simulink model "kalman_direction_updater"  (R2014a)
settings: Solver=FixedStepDiscrete  StartTime=0.0  StopTime=t_sim  FixedStep=t_step  RelTol=1e-3
undefined symbols (not defined in the file): omega_B
libraries: lib_gyro_fusion x7, vrlib x1
settings Model: Creator=kirill  LastModifiedBy=kirill

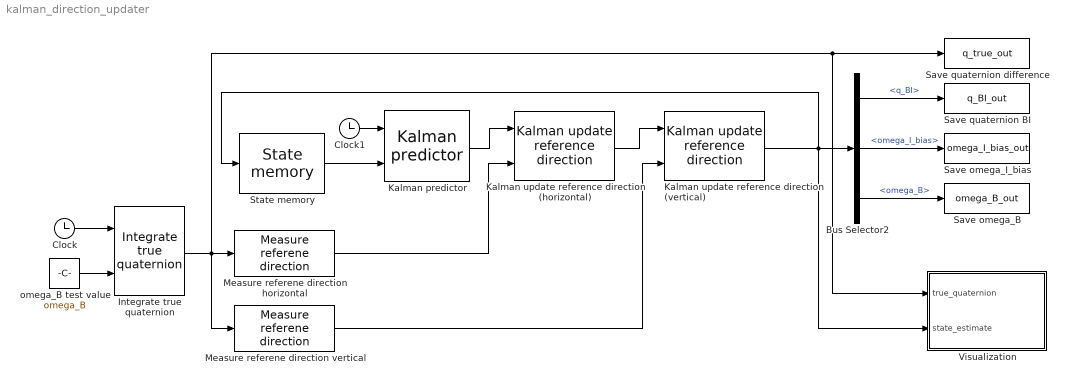
== system kalman_direction_updater ==
  Bus Selector2 : BusSelector  OutputSignals=q_BI,omega_I_bias,omega_B
  Clock : Clock
  Clock1 : Clock
  Integrate true quaternion : lib_gyro_fusion/Integrate true quaternion  q_BI_init=q_init
  Kalman predictor : lib_gyro_fusion/Kalman predictor  q_noise=q_noise  omega_B_noise=omega_B_noise  omega_I_bias_noise=omega_bias_I_noise
  Kalman update reference direction (horizontal) : lib_gyro_fusion/Kalman update reference direction
  Kalman update reference direction (vertical) : lib_gyro_fusion/Kalman update reference direction
  Measure referene direction horizontal : lib_gyro_fusion/Measure referene direction  ref_direction=horizontal_direction  measurement_noise_power=horizontal_direction_noise_power  measurement_sample_rate=t_step  source_seeds=horizontal_direction_seeds  R_direction=horizontal_direction_R
  Measure referene direction vertical : lib_gyro_fusion/Measure referene direction  ref_direction=vertical_direction  measurement_noise_power=vertical_direction_noise_power  measurement_sample_rate=t_step  source_seeds=vertical_direction_seeds  R_direction=vertical_direction_R
  Save omega_B : ToWorkspace  VariableName=omega_B_out  SaveFormat=Timeseries  SampleTime=-1
  Save omega_I_bias : ToWorkspace  VariableName=omega_I_bias_out  SaveFormat=Timeseries  SampleTime=-1
  Save quaternion BI : ToWorkspace  VariableName=q_BI_out  SaveFormat=Timeseries  SampleTime=-1
  Save quaternion difference : ToWorkspace  VariableName=q_true_out  SaveFormat=Timeseries  SampleTime=-1
  State memory : lib_gyro_fusion/State memory  q_BI_init=[1; 0; 0; 0]  omega_B_init=[0; 0; 0]  omega_I_bias_init=[0; 0; 0]  P_full_init=eye(9)
  Visualization : Subsystem
  omega_B test value : Constant  Value=omega_B
  wires:
  State memory/1 -> Kalman predictor/2
  Clock/1 -> Integrate true quaternion/1
  Integrate true quaternion/1 -> Measure referene direction horizontal/1, Measure referene direction vertical/1, Visualization/1(true_quaternion), Save quaternion difference/1
  omega_B test value/1 -> Integrate true quaternion/2
  Bus Selector2/2 -> Save omega_I_bias/1  "<omega_I_bias>"
  Bus Selector2/3 -> Save omega_B/1  "<omega_B>"
  Kalman update reference direction (vertical)/1 -> State memory/1, Visualization/2(state_estimate), Bus Selector2/1
  Bus Selector2/1 -> Save quaternion BI/1  "<q_BI>"
  Clock1/1 -> Kalman predictor/1
  Kalman predictor/1 -> Kalman update reference direction (horizontal)/1
  Measure referene direction horizontal/1 -> Kalman update reference direction (horizontal)/2
  Kalman update reference direction (horizontal)/1 -> Kalman update reference direction (vertical)/1
  Measure referene direction vertical/1 -> Kalman update reference direction (vertical)/2

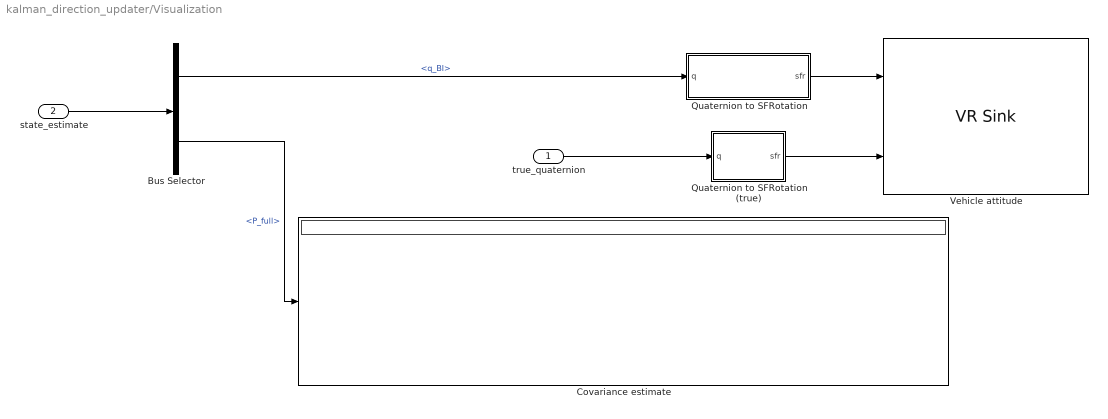
== system kalman_direction_updater/Visualization ==
  true_quaternion : Inport
  state_estimate : Inport  Port=2
  Bus Selector : BusSelector  OutputSignals=q_BI,P_full
  Covariance estimate : Display
  Quaternion to SFRotation : MATLAB Function  TreatAsAtomicUnit=on
  Quaternion to SFRotation (true) : MATLAB Function  TreatAsAtomicUnit=on
  Vehicle attitude : vrlib/VR Sink  InstantiateOnLoad=on  SampleTime=0.1  ViewEnable=on  RemoteChange=off  RemoteView=off  FieldsWritten=Estimated_car.rotation.4.1.1.double#True_car.rotation.4.1.1.double  WorldFileName=ins.wrl  AutoView=off  VideoDimensions=[]  AllowVariableSize=off
  wires:
  Bus Selector/2 -> Covariance estimate/1  "<P_full>"
  state_estimate/1 -> Bus Selector/1
  Bus Selector/1 -> Quaternion to SFRotation/1(q)  "<q_BI>"
  Quaternion to SFRotation (true)/1(sfr) -> Vehicle attitude/2
  Quaternion to SFRotation/1(sfr) -> Vehicle attitude/1
  true_quaternion/1 -> Quaternion to SFRotation (true)/1(q)

== matlab function kalman_direction_updater/Visualization/Quaternion to SFRotation ==
  data: q input; sfr output
function sfr = quaternion2rotation(q)
%#codegen

sfr = zeros(size(q));
sfr(1:3) = q(2:4);
sfr(4) = acos(q(1));

== matlab function kalman_direction_updater/Visualization/Quaternion to SFRotation (true) ==
  data: q input; sfr output
function sfr = quaternion2rotation(q)
%#codegen

sfr = zeros(size(q));
sfr(1:3) = q(2:4);
sfr(4) = acos(q(1));
